simulink model "Tracking_with_dynamic_lin"  (R2023a)
settings: Solver=ode1  StartTime=0  StopTime=40  FixedStep=0.01  RelTol=1e-3
PostLoadFcn:
  | p=1:640; % pixels from left to right
  | 
  | Obtained_angles=(320-p).*(57/640)*pi./180;  % Kinect's horizontal FOV = 57 degrees
  | 
  | S=400; % S = Size of the 2D Map matrix... the highet S is the higher resolution we would end up with - %00 might be high for Embedded computing
values from neighbouring files (symbols this model uses):
  parameters = [R,D,omega,Ts,db,vm]    [Mian_tracking_using_dyn_lin_Quanser.m]
  Q0 = double(Q)    [worse_case_NB.m]
  R = 0.035    [Mian_tracking_using_dyn_lin_Quanser.m]
  T = [R/2 R/2 ... (first row only)    [Mian_tracking_using_dyn_lin_Quanser.m]
  X0 = [-0.25 -0.75 0]'    [Mian_tracking_using_dyn_lin_Quanser.m]
undefined symbols (not defined in the file or in its folder): HIL, p1, p2, qc_get_step_size, Video3D
libraries: quarc_library x8
settings Model: ExtModeTrigDuration=2  Creator=drmadill  LastModifiedBy=Ferna
settings SolverCC: AlgebraicLoopSolver=TrustRegion
settings DebuggingCC: UnderspecifiedInitializationDetection=Classic  MergeDetectMultiDrivingBlocksExec=none  UnconnectedInputMsg=warning  UnconnectedOutputMsg=warning  UnconnectedLineMsg=warning
settings ModelReferenceCC: EnableRefExpFcnMdlSchedulingChecks=on  PropagateSignalLabelsOutOfModel=off

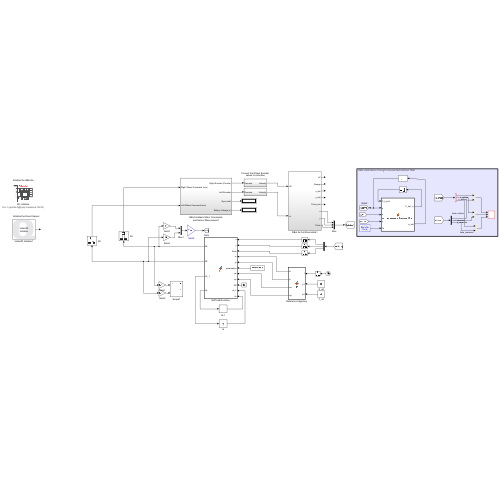
[thumbnail: Simulink's stored preview of the top-level diagram]
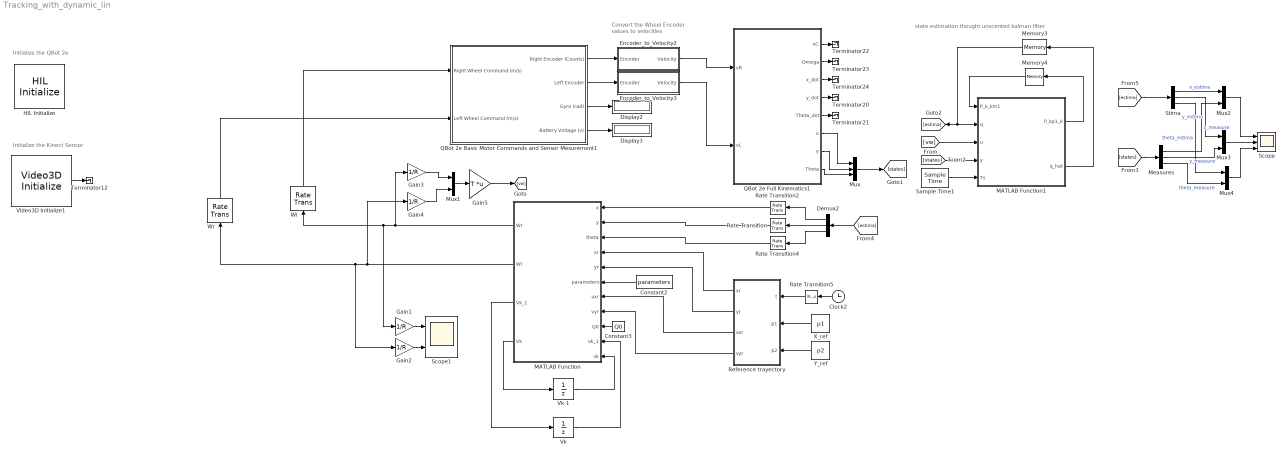
== system Tracking_with_dynamic_lin ==
  note: Initialize the QBot 2e
  note: Initialize the Kinect Sensor
  note: Convert the Wheel Encoder
      | values to velocities
  note: state estimation thought unscented kalman filter
  Clock2 : Clock
  Constant2 : Constant  Value=parameters
  Constant3 : Constant  Value=Q0
  Demux2 : Demux  Outputs=3
  Display2 : Display
  Display3 : Display
  Encoder_to_Velocity2 : Subsystem
  Encoder_to_Velocity3 : Subsystem
  Gain{1..4} (4 alike) : Gain  Gain=1/R
  Gain5 : Gain  Gain=T  Multiplication=Matrix(K*u)
  HIL Initialize : quarc_library/Data Acquisition/Generic/Configuration/HIL Initialize  Priority=-99  object_name=HIL-1  board_type=qbot2e  board_number=0@tcpip://localhost:18910  board_options=pwm0_en=1;pwm0_pin=12;pwm1_en=1;pwm1_pin=13;  exclusive=off  active=on  hardware_clocks=[]  clock_modes=[]  initial_clock_frequencies=[]  set_clock_params_at_start=off  set_clock_params_at_switch_in=off  set_clock_frequencies_at_start=off  set_clock_frequencies_at_switch_in=off  analog_input_channels=[0:5]  analog_input_configurations=[]  analog_input_maximums=[16.5 3.3 3.3 3.3 3.3 3.3]  analog_input_minimums=[0 0 0 0 0 0]  set_analog_input_params_at_start=off  set_analog_input_params_at_switch_in=off  analog_output_channels=[]  analog_output_maximums=[]  analog_output_minimums=[]  initial_analog_outputs=[]  final_analog_outputs=[]  watchdog_analog_outputs=[]  set_analog_output_params_at_start=off  set_analog_output_params_at_switch_in=off  set_analog_outputs_at_start=off  set_analog_outputs_at_switch_in=off  set_analog_outputs_at_terminate=off  set_analog_outputs_at_switch_out=off  set_analog_outputs_on_watchdog=off  digital_input_channels=[28:58]  digital_output_channels=[28:31]  digital_output_configuration=[]  initial_digital_outputs=[0]  final_digital_outputs=[0]  watchdog_digital_outputs=[]  set_digital_output_params_at_start=off  set_digital_output_params_at_switch_in=off  set_digital_outputs_at_start=on  set_digital_outputs_at_switch_in=off  set_digital_outputs_at_terminate=on  set_digital_outputs_at_switch_out=off  set_digital_outputs_on_watchdog=off  encoder_channels=[0:1]  quadrature=[4]  encoder_filter_frequency=[]  initial_encoder_counts=[0]  set_encoder_params_at_start=on  set_encoder_params_at_switch_in=off  set_encoder_counts_at_start=on  set_encoder_counts_at_switch_in=off  pwm_channels=[0:1]  pwm_modes=0  pwm_frequency=100e6 / 4095  pwm_configuration=[0]  pwm_alignment=[0]  pwm_polarity=[1]  pwm_leading_deadband=[]  pwm_trailing_deadband=[]  initial_pwm_outputs=[0]  final_pwm_outputs=[0]  watchdog_pwm_outputs=[]  set_pwm_params_at_start=on  set_pwm_params_at_switch_in=off  set_pwm_outputs_at_start=on  set_pwm_outputs_at_switch_in=off  set_pwm_outputs_at_terminate=on  set_pwm_outputs_at_switch_out=off  set_pwm_outputs_on_watchdog=off  other_output_channels=[2000:2001 14000 16000]  initial_other_outputs=[0 0 0 7]  final_other_outputs=[0 0 0 7]  watchdog_other_outputs=[]  set_other_outputs_at_start=on  set_other_outputs_at_switch_in=off  set_other_outputs_at_terminate=on  set_other_outputs_at_switch_out=off  set_other_outputs_on_watchdog=off
  MATLAB Function : MATLAB Function  TreatAsAtomicUnit=on
  MATLAB Function1 : MATLAB Function  TreatAsAtomicUnit=on
  Measures : Demux  Outputs=3
  Memory3 : Memory  InitialCondition=X0
  Memory4 : Memory  InitialCondition=1e-6*eye(3)
  Mux : Mux  Inputs=3
  Mux{1..4} (4 alike) : Mux  Inputs=2
  QBot 2e Basic Motor Commands and Sensor Mesurement1 : Subsystem
  QBot 2e Full Kinematics1 : Subsystem
  Rate Transition{,2,4..5} (4 alike) : RateTransition  OutPortSampleTime=Ts
  Reference trayectory : MATLAB Function  TreatAsAtomicUnit=on
  Sample Time1 : quarc_library/Sources/Time/Sample Time  Priority=-99  sample_time=Ts
  Scope : Scope  NumInputPorts=3
  Scope1 : Scope  NumInputPorts=2
  Stima : Demux  Outputs=3
  Terminator{12,20..24} (6 alike) : Terminator
  Video3D Initialize1 : quarc_library/Multimedia/Video3D Initialize  object_name=Video3D-1  source=Device  identifier=0@tcpip://localhost:18911  file=sample.bag  sample_time=qc_get_step_size * ceil(0.033 / qc_get_step_size)  active=on
  Vk : UnitDelay  InitialCondition=0.01  SampleTime=-1  HasFrameUpgradeWarning=on
  Vk-1 : UnitDelay  InitialCondition=0.01  SampleTime=-1  HasFrameUpgradeWarning=on
  Wl : RateTransition
  Wr : RateTransition
  X_ref : Constant  Value=p1
  Y_ref : Constant  Value=p2
  wires:
  Video3D Initialize1/1 -> Terminator12/1
  QBot 2e Basic Motor Commands and Sensor Mesurement1/1(Right Encoder (Counts)) -> Encoder_to_Velocity2/1(Encoder)
  QBot 2e Basic Motor Commands and Sensor Mesurement1/2(Left Encoder) -> Encoder_to_Velocity3/1(Encoder)
  QBot 2e Basic Motor Commands and Sensor Mesurement1/4(Battery Voltage (v)) -> Display3/1
  QBot 2e Basic Motor Commands and Sensor Mesurement1/3(Gyro (rad)) -> Display2/1
  QBot 2e Full Kinematics1/4(y_dot) -> Terminator20/1
  QBot 2e Full Kinematics1/3(x_dot) -> Terminator24/1
  Encoder_to_Velocity2/1(Velocity) -> QBot 2e Full Kinematics1/1(vR)
  QBot 2e Full Kinematics1/5(Theta_dot) -> Terminator21/1
  QBot 2e Full Kinematics1/2(Omega) -> Terminator23/1
  QBot 2e Full Kinematics1/1(vC) -> Terminator22/1
  Encoder_to_Velocity3/1(Velocity) -> QBot 2e Full Kinematics1/2(vL)
  Rate Transition2/1 -> MATLAB Function/1(x)
  Rate Transition4/1 -> MATLAB Function/3(theta)
  MATLAB Function/1(Wr) -> Gain3/1, Wl/1, Gain1/1
  Rate Transition5/1 -> Reference trayectory/1(t)
  X_ref/1 -> Reference trayectory/2(p1)
  Y_ref/1 -> Reference trayectory/3(p2)
  Constant2/1 -> MATLAB Function/6(parameters)
  Rate Transition/1 -> MATLAB Function/2(y)
  Reference trayectory/1(xr) -> MATLAB Function/4(xr)
  Reference trayectory/2(yr) -> MATLAB Function/5(yr)
  MATLAB Function/2(Wl) -> Gain4/1, Wr/1, Gain2/1
  Wr/1 -> QBot 2e Basic Motor Commands and Sensor Mesurement1/2(Left Wheel Command (m/s))
  Wl/1 -> QBot 2e Basic Motor Commands and Sensor Mesurement1/1(Right Wheel Command (m/s))
  Gain1/1 -> Scope1/1
  Gain2/1 -> Scope1/2
  MATLAB Function/3(Vk_1) -> Vk/1
  MATLAB Function/4(Vk) -> Vk-1/1
  Vk/1 -> MATLAB Function/10(vk_1)
  Vk-1/1 -> MATLAB Function/11(vk)
  Reference trayectory/3(vxr) -> MATLAB Function/7(vxr)
  Reference trayectory/4(vyr) -> MATLAB Function/8(vyr)
  Constant3/1 -> MATLAB Function/9(Q0)
  Measures/1 -> Mux2/2  "x_measure"
  Mux3/1 -> Scope/2
  [vw] -> MATLAB Function1/3(u)
  Mux4/1 -> Scope/3
  Stima/3 -> Mux4/1  "theta_estima"
  MATLAB Function1/1(P_kp1_k) -> Memory4/1
  Measures/3 -> Mux4/2  "theta_measure"
  MATLAB Function1/2(q_hat) -> Memory3/1
  Memory4/1 -> MATLAB Function1/1(P_k_km1)
  Memory3/1 -> MATLAB Function1/2(q), [estima]
  [estima] -> Stima/1
  [states] -> Measures/1
  Measures/2 -> Mux3/2  "y_measure"
  Stima/1 -> Mux2/1  "x_estima"
  Stima/2 -> Mux3/1  "y_estima"
  Sample Time1/1 -> MATLAB Function1/5(Ts)
  Mux2/1 -> Scope/1
  [states] -> MATLAB Function1/4(y)
  Mux/1 -> [states]
  QBot 2e Full Kinematics1/6(x) -> Mux/1
  QBot 2e Full Kinematics1/7(y) -> Mux/2
  QBot 2e Full Kinematics1/8(Theta) -> Mux/3
  [estima] -> Demux2/1
  Demux2/1 -> Rate Transition2/1
  Demux2/2 -> Rate Transition/1
  Demux2/3 -> Rate Transition4/1
  Gain4/1 -> Mux1/2
  Gain5/1 -> [vw]
  Gain3/1 -> Mux1/1
  Mux1/1 -> Gain5/1
  Clock2/1 -> Rate Transition5/1

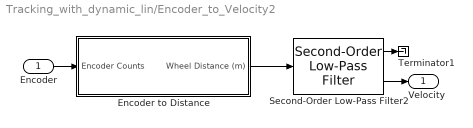
== system Tracking_with_dynamic_lin/Encoder_to_Velocity2 ==
  Encoder : Inport
  Encoder to Distance : Subsystem
  Second-Order Low-Pass Filter2 : quarc_library/Continuous/Second-Order Low-Pass Filter  params_source=Internal (dialog parameters)  input_width=10  input_zeta=1  input_init=0
  Terminator1 : Terminator
  Velocity : Outport  VectorParamsAs1DForOutWhenUnconnected=off
  wires:
  Second-Order Low-Pass Filter2/1 -> Terminator1/1
  Encoder to Distance/1(Wheel Distance (m)) -> Second-Order Low-Pass Filter2/1
  Encoder/1 -> Encoder to Distance/1(Encoder Counts)
  Second-Order Low-Pass Filter2/2 -> Velocity/1

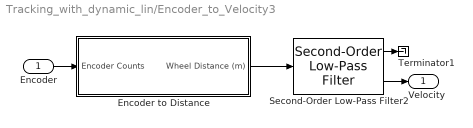
== system Tracking_with_dynamic_lin/Encoder_to_Velocity3 ==
  Encoder : Inport
  Encoder to Distance : Subsystem
  Second-Order Low-Pass Filter2 : quarc_library/Continuous/Second-Order Low-Pass Filter  params_source=Internal (dialog parameters)  input_width=10  input_zeta=1  input_init=0
  Terminator1 : Terminator
  Velocity : Outport  VectorParamsAs1DForOutWhenUnconnected=off
  wires:
  Second-Order Low-Pass Filter2/2 -> Velocity/1
  Encoder/1 -> Encoder to Distance/1(Encoder Counts)
  Encoder to Distance/1(Wheel Distance (m)) -> Second-Order Low-Pass Filter2/1
  Second-Order Low-Pass Filter2/1 -> Terminator1/1

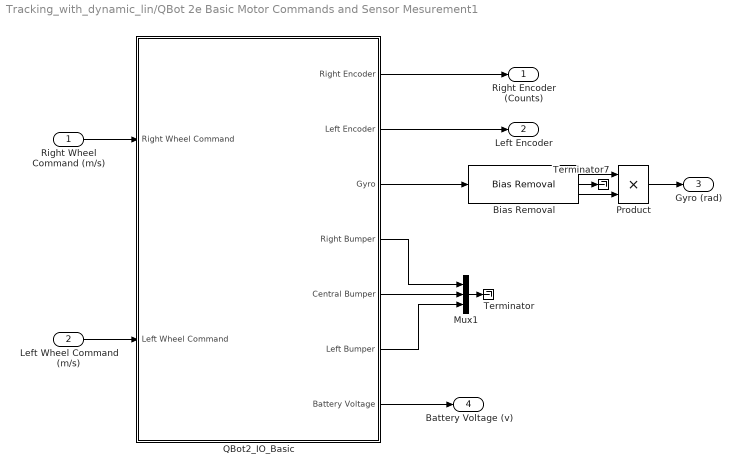
== system Tracking_with_dynamic_lin/QBot 2e Basic Motor Commands and Sensor Mesurement1 ==
  Right Wheel Command (m/s) : Inport
  Left Wheel Command (m/s) : Inport  Port=2
  Bias Removal : quarc_library/Discrete/Bias Removal  start_time=3  end_time=4  switch_id=0  sample_time=qc_get_step_size
      settings: SourceProductName=QUARC Targets
  Mux1 : Mux  Inputs=3
  Product : Product  RndMeth=Zero
  QBot2_IO_Basic : Subsystem
  Terminator : Terminator
  Terminator7 : Terminator
  Right Encoder (Counts) : Outport  VectorParamsAs1DForOutWhenUnconnected=off
  Left Encoder : Outport  Port=2  VectorParamsAs1DForOutWhenUnconnected=off
  Gyro (rad) : Outport  Port=3  VectorParamsAs1DForOutWhenUnconnected=off
  Battery Voltage (v) : Outport  Port=4  VectorParamsAs1DForOutWhenUnconnected=off
  wires:
  QBot2_IO_Basic/4(Right Bumper) -> Mux1/1
  QBot2_IO_Basic/5(Central Bumper) -> Mux1/2
  QBot2_IO_Basic/6(Left Bumper) -> Mux1/3
  Right Wheel Command (m/s)/1 -> QBot2_IO_Basic/1(Right Wheel Command)
  Left Wheel Command (m/s)/1 -> QBot2_IO_Basic/2(Left Wheel Command)
  QBot2_IO_Basic/1(Right Encoder) -> Right Encoder (Counts)/1
  QBot2_IO_Basic/2(Left Encoder) -> Left Encoder/1
  QBot2_IO_Basic/7(Battery Voltage) -> Battery Voltage (v)/1
  Bias Removal/2 -> Terminator7/1
  Bias Removal/1 -> Product/1
  Bias Removal/3 -> Product/2
  Product/1 -> Gyro (rad)/1
  QBot2_IO_Basic/3(Gyro) -> Bias Removal/1
  Mux1/1 -> Terminator/1

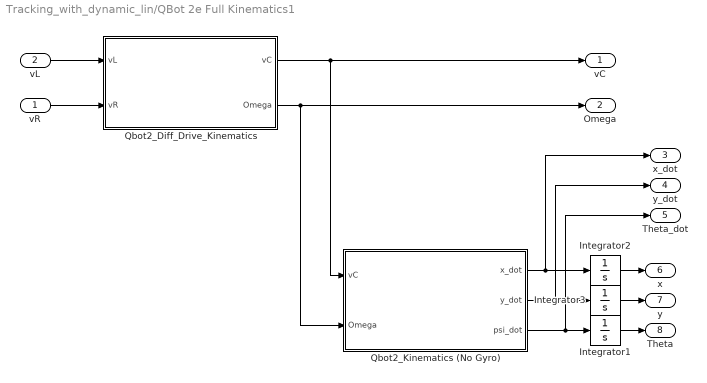
== system Tracking_with_dynamic_lin/QBot 2e Full Kinematics1 ==
  vR : Inport
  vL : Inport  Port=2
  Integrator1 : Integrator  InitialCondition=X0(3)
  Integrator2 : Integrator  InitialCondition=X0(1)
  Integrator3 : Integrator  InitialCondition=X0(2)
  Qbot2_Diff_Drive_Kinematics : Subsystem
  Qbot2_Kinematics (No Gyro) : Subsystem
  vC : Outport  VectorParamsAs1DForOutWhenUnconnected=off
  Omega : Outport  Port=2  VectorParamsAs1DForOutWhenUnconnected=off
  x_dot : Outport  Port=3  VectorParamsAs1DForOutWhenUnconnected=off
  y_dot : Outport  Port=4  VectorParamsAs1DForOutWhenUnconnected=off
  Theta_dot : Outport  Port=5  VectorParamsAs1DForOutWhenUnconnected=off
  x : Outport  Port=6  VectorParamsAs1DForOutWhenUnconnected=off
  y : Outport  Port=7  VectorParamsAs1DForOutWhenUnconnected=off
  Theta : Outport  Port=8  VectorParamsAs1DForOutWhenUnconnected=off
  wires:
  Integrator1/1 -> Theta/1
  Qbot2_Kinematics (No Gyro)/3(psi_dot) -> Theta_dot/1, Integrator1/1
  Qbot2_Kinematics (No Gyro)/1(x_dot) -> x_dot/1, Integrator2/1
  Qbot2_Kinematics (No Gyro)/2(y_dot) -> y_dot/1, Integrator3/1
  Qbot2_Diff_Drive_Kinematics/1(vC) -> Qbot2_Kinematics (No Gyro)/1(vC), vC/1
  vL/1 -> Qbot2_Diff_Drive_Kinematics/1(vL)
  vR/1 -> Qbot2_Diff_Drive_Kinematics/2(vR)
  Integrator2/1 -> x/1
  Integrator3/1 -> y/1
  Qbot2_Diff_Drive_Kinematics/2(Omega) -> Qbot2_Kinematics (No Gyro)/2(Omega), Omega/1

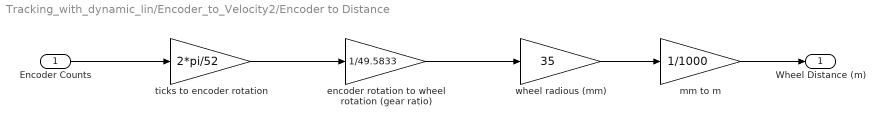
== system Tracking_with_dynamic_lin/Encoder_to_Velocity2/Encoder to Distance ==
  Encoder Counts : Inport
  " encoder rotation to wheel rotation (gear ratio)" : Gain  Gain=1/49.5833
  mm to m : Gain  Gain=1/1000
  ticks to encoder rotation : Gain  Gain=2*pi/52
  wheel radious (mm) : Gain  Gain=35
  Wheel Distance (m) : Outport  VectorParamsAs1DForOutWhenUnconnected=off
  wires:
  Encoder Counts/1 -> ticks to encoder rotation/1
  ticks to encoder rotation/1 -> " encoder rotation to wheel rotation (gear ratio)"/1
  " encoder rotation to wheel rotation (gear ratio)"/1 -> wheel radious (mm)/1
  wheel radious (mm)/1 -> mm to m/1
  mm to m/1 -> Wheel Distance (m)/1

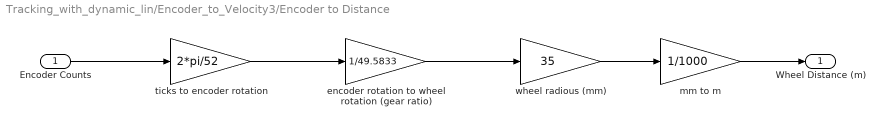
== system Tracking_with_dynamic_lin/Encoder_to_Velocity3/Encoder to Distance ==
  Encoder Counts : Inport
  " encoder rotation to wheel rotation (gear ratio)" : Gain  Gain=1/49.5833
  mm to m : Gain  Gain=1/1000
  ticks to encoder rotation : Gain  Gain=2*pi/52
  wheel radious (mm) : Gain  Gain=35
  Wheel Distance (m) : Outport  VectorParamsAs1DForOutWhenUnconnected=off
  wires:
  mm to m/1 -> Wheel Distance (m)/1
  wheel radious (mm)/1 -> mm to m/1
  " encoder rotation to wheel rotation (gear ratio)"/1 -> wheel radious (mm)/1
  ticks to encoder rotation/1 -> " encoder rotation to wheel rotation (gear ratio)"/1
  Encoder Counts/1 -> ticks to encoder rotation/1

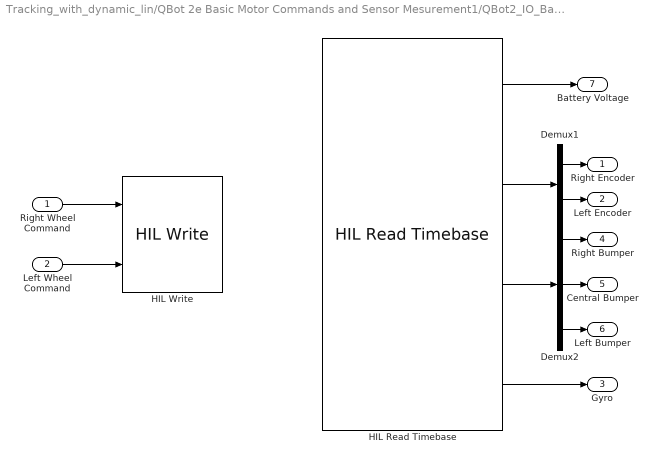
== system Tracking_with_dynamic_lin/QBot 2e Basic Motor Commands and Sensor Mesurement1/QBot2_IO_Basic ==
  Right Wheel Command : Inport
  Left Wheel Command : Inport  Port=2
  Demux1 : Demux  Outputs=2
  Demux2 : Demux  Outputs=3
  HIL Read Timebase : quarc_library/Data Acquisition/Generic/Timebases/HIL Read Timebase  object_name=HIL-1  clock=0  analog_channels=0  encoder_channels=0:1  digital_channels=28:30  other_channels=1002  active=on  vector_output=on  data_type_mode=Inherit via back propagation  encoder_data_type=double  digital_data_type=boolean  overflow_mode=Synchronize (for simulated cards only)  samples_in_buffer=1+0*max(ceil(1/qc_get_step_size), 1)
  HIL Write : quarc_library/Data Acquisition/Generic/Immediate I//O/HIL Write  object_name=HIL-1  analog_channels=[]  pwm_channels=[]  digital_channels=[]  other_channels=[2000:2001]  sample_time=-1  active=on  vector_input=off
  Right Encoder : Outport  VectorParamsAs1DForOutWhenUnconnected=off
  Left Encoder : Outport  Port=2  VectorParamsAs1DForOutWhenUnconnected=off
  Gyro : Outport  Port=3  VectorParamsAs1DForOutWhenUnconnected=off
  Right Bumper : Outport  Port=4  VectorParamsAs1DForOutWhenUnconnected=off
  Central Bumper : Outport  Port=5  VectorParamsAs1DForOutWhenUnconnected=off
  Left Bumper : Outport  Port=6  VectorParamsAs1DForOutWhenUnconnected=off
  Battery Voltage : Outport  Port=7  VectorParamsAs1DForOutWhenUnconnected=off
  wires:
  HIL Read Timebase/1 -> Battery Voltage/1
  HIL Read Timebase/3 -> Demux2/1
  HIL Read Timebase/4 -> Gyro/1
  Demux1/1 -> Right Encoder/1
  Demux1/2 -> Left Encoder/1
  Right Wheel Command/1 -> HIL Write/1
  Left Wheel Command/1 -> HIL Write/2
  HIL Read Timebase/2 -> Demux1/1
  Demux2/1 -> Right Bumper/1
  Demux2/2 -> Central Bumper/1
  Demux2/3 -> Left Bumper/1

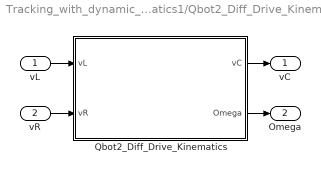
== system Tracking_with_dynamic_lin/QBot 2e Full Kinematics1/Qbot2_Diff_Drive_Kinematics ==
  vL : Inport
  vR : Inport  Port=2
  Qbot2_Diff_Drive_Kinematics : MATLAB Function  TreatAsAtomicUnit=on
  vC : Outport  VectorParamsAs1DForOutWhenUnconnected=off
  Omega : Outport  Port=2  VectorParamsAs1DForOutWhenUnconnected=off
  wires:
  vL/1 -> Qbot2_Diff_Drive_Kinematics/1(vL)
  Qbot2_Diff_Drive_Kinematics/1(vC) -> vC/1
  vR/1 -> Qbot2_Diff_Drive_Kinematics/2(vR)
  Qbot2_Diff_Drive_Kinematics/2(Omega) -> Omega/1

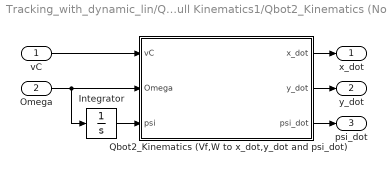
== system Tracking_with_dynamic_lin/QBot 2e Full Kinematics1/Qbot2_Kinematics (No Gyro) ==
  vC : Inport
  Omega : Inport  Port=2
  Integrator : Integrator
  Qbot2_Kinematics (Vf,W to x_dot,y_dot and psi_dot) : MATLAB Function  TreatAsAtomicUnit=on
  x_dot : Outport  VectorParamsAs1DForOutWhenUnconnected=off
  y_dot : Outport  Port=2  VectorParamsAs1DForOutWhenUnconnected=off
  psi_dot : Outport  Port=3  VectorParamsAs1DForOutWhenUnconnected=off
  wires:
  Qbot2_Kinematics (Vf,W to x_dot,y_dot and psi_dot)/3(psi_dot) -> psi_dot/1
  Integrator/1 -> Qbot2_Kinematics (Vf,W to x_dot,y_dot and psi_dot)/3(psi)
  vC/1 -> Qbot2_Kinematics (Vf,W to x_dot,y_dot and psi_dot)/1(vC)
  Qbot2_Kinematics (Vf,W to x_dot,y_dot and psi_dot)/1(x_dot) -> x_dot/1
  Omega/1 -> Integrator/1, Qbot2_Kinematics (Vf,W to x_dot,y_dot and psi_dot)/2(Omega)
  Qbot2_Kinematics (Vf,W to x_dot,y_dot and psi_dot)/2(y_dot) -> y_dot/1

== matlab function Tracking_with_dynamic_lin/MATLAB Function1 ==
  data: P_k_km1 input; P_kp1_k output; q input; u input; q_hat output; y input; Ts input
function [P_kp1_k,q_hat]= my_unscented_kalman_filter(P_k_km1,q,u,y,Ts)
Q=1e-6*eye(3);
R=1e-6*eye(3);
alpha=0.9; beta=2; kappa=0;
%Calculate the Sigma points
M=3;
c=alpha^2*(M+kappa);
q_hat_i=zeros(M,2*M+1);
q_hat_i(:,1)=q;
Delta_x=real(sqrtm(c*P_k_km1));
for i=1:M
    q_hat_i(:,i+1)=q+Delta_x(:,i);
    q_hat_i(:,i+1+M)=q-Delta_x(:,i);
end
%Output of the sigma points
y_hat_i=q_hat_i(1:3,:);
%predicted measurement at time k
W_M=zeros(1,2*M+1);
W_M(1)=1-(M/(alpha^2*(M+kappa)));
W_M(2:2*M+1)=(1/(2*alpha^2*(M+kappa)));
y_k=zeros(3,1);
for i=1:2*M+1
    y_k=y_k+W_M(i)*y_hat_i(:,i);
end
%Estimate of the covariance of predicted measurement
W_c=zeros(1,2*M+1);
W_c(1)=(2-alpha^2+beta)-(M/(alpha^2*(M+kappa)));
W_c(2:2*M+1)=(1/(2*alpha^2*(M+kappa)));
P_y=zeros(3,3);
for i=1:2*M+1
    P_y=P_y+W_c(i)*(y_hat_i(:,i)-y_k)*(y_hat_i(:,i)-y_k)'+R;
end
%%Estimate of the cross-covariance between predicted x and y
P_xy=zeros(M,3);
for i=1:2*M+1
    P_xy=P_xy+(1/(2*alpha^2*(M+kappa)))*(q_hat_i(:,i)-q)*(y_hat_i(:,i)-y_k)';
end
%Kalman gain
K=P_xy/(P_y);
q_k_k = q+K*(y-y_k);
P_k_k = P_k_km1 -K*P_y*K';
% State prediction and state estimation error covariance
q_hat_i_k_k=zeros(M,2*M+1);
q_hat_i_k_k(:,1)=q_k_k;
Delta_x=real(sqrtm(c*P_k_k));
for i=1:M
    q_hat_i_k_k(:,i+1)=q_k_k+Delta_x(:,i);
    q_hat_i_k_k(:,i+1+M)=q_k_k-Delta_x(:,i);
end
%Predicted state for each sigma point
q_hat_kp1_k=zeros(M,2*M+1);
for i=1:2*M+1
    q_hat_kp1_k(:,i)=q_hat_i_k_k(:,i)+Ts*[cos(q_hat_i_k_k(3,i)) 0;
        sin(q_hat_i_k_k(3,i)) 0;
        0          1]*u;
end
%Predicted state k+1 at time k
q_hat=zeros(M,1);
for i=1:2*M+1
    q_hat=q_hat + W_M(i)*q_hat_kp1_k(:,i);
end
%Covariance of the predicted state
P_kp1_k=zeros(M,M);
for i=1:2*M+1
    P_kp1_k=P_kp1_k+W_c(i)*(q_hat_kp1_k(:,i)-q_hat)*(q_hat_kp1_k(:,i)-q_hat)'+Q;
end
end

== matlab function Tracking_with_dynamic_lin/QBot 2e Full Kinematics1/Qbot2_Diff_Drive_Kinematics/Qbot2_Diff_Drive_Kinematics ==
  data: vL input; vC output; vR input; Omega output
function [vC,Omega] = fcn(vL,vR)
%#codegen

d= 0.235;

vC=0.5*(vL+vR);
Omega=(1/d)*(vR-vL);

== matlab function Tracking_with_dynamic_lin/QBot 2e Full Kinematics1/Qbot2_Kinematics (No Gyro)/Qbot2_Kinematics (Vf,W to x_dot,y_dot and psi_dot) ==
  data: vC input; x_dot output; Omega input; y_dot output; psi input; psi_dot output
function [x_dot,y_dot,psi_dot] = fcn(vC,Omega,psi)
%#codegen


x_dot=cos(psi)*vC;
y_dot=sin(psi)*vC;
psi_dot= Omega;

== matlab function Tracking_with_dynamic_lin/MATLAB Function ==
  data: x input; Wr output; y input; theta input; Wl output; Vk_1 output; Vk output; xr input; yr input; parameters input; vxr input; vyr input; Q0 input; vk_1 input; vk input
function [Wr, Wl, Vk_1, Vk] = fcn(x,y,theta, xr, yr, parameters, vxr, vyr, Q0, vk_1, vk)
%#codegen
coder.extrinsic("RHC_Dy_lin_mincx")
R=parameters(1);        % radius od wheels [m]
D=parameters(2);      % distance between the two wheels [m]
omega=parameters(3);   % max angular velocity [rad/s] 
Ts=parameters(4);      % sampling time [s]
db=parameters(5);         % distance point b [m]
Vm=parameters(6);         % distance point b [m]

uk=zeros(1,2)';

A=[1 0 Ts 0;
    0 1 0 Ts;
    0 0 1 0;
    0 0 0 1];

B=[(Ts*Ts)/2 0;
    0 (Ts*Ts)/2;
    Ts 0;
    0 Ts];

Hd=[-1/omega 0 1/omega 0;
    0 -1/omega 0 1/omega]';

T=[R/2 R/2;     % diff drive to unicycle
    R/D -R/D];
Tinv=inv(T);

Qbd=[db*db 0  % vision radius 
    0 db*db];

Hu=Hd*Tinv;

HTs=[Ts 0;
     0 1];


Qe=[100 0 0 0;
    0 100 0 0;
    0 0 0 0;
    0 0 0 0];

rho=0.0001;
Qu=rho*eye(2);

% Err = [x;y;vk*cos(theta);vk*sin(theta)]-[xr;yr;vxr;vyr];
Err = [x;y;vk*cos(theta);vk*sin(theta)]-[xr;yr;0;0];

Tfl = [cos(theta) -vk*sin(theta);
       sin(theta) vk*cos(theta)];

H_theta_v = Hu*HTs*inv(Tfl);
nk=[vk_1/Ts;0];
Q_str=zeros(4,4);
Y_str=zeros(2,4);
[Q_str,Y_str] = RHC_Dy_lin_mincx(Err,A,B,H_theta_v,Qe,Qu,Q0);

uk=Y_str*inv(Q_str)*Err-Tfl*nk;
u=inv(Tfl)*uk;         % aceleration and angular velocity
acel=u(1);        % take the aceleration
vel=acel*Ts+vk_1; % back derivate aproximation to take the velocity
 
% v(k-1) equal to previus v(k) equal to current
Vk_1=vk;
Vk=vel;
    

vw=[vk;u(2)];   % angular right and left velocities      
wrwl=Tinv*vw;
wr=wrwl(1); 
wl=wrwl(2);

Wr=wr*R;
Wl=wl*R;

== matlab function Tracking_with_dynamic_lin/Reference trayectory ==
  data: t input; xr output; yr output; p1 input; p2 input; vxr output; vyr output
function [xr,yr,vxr,vyr] = fcn(t,p1,p2)

xr=polyval(p1,t);
yr=polyval(p2,t);

xrd=polyder(p1);
yrd=polyder(p2);

vxr=polyval(xrd,t);
vyr=polyval(yrd,t);
